simulink model "hethong_RR1"  (R2023a)
settings: Solver=FixedStepDiscrete  StartTime=0.0  StopTime=0  FixedStep=T_sample  RelTol=1e-3  EnableMultiTasking=on
values from neighbouring files (symbols this model uses):
  A = A_d    [GiaiBT_compactversion.m]    (also in KhoaModified_of_RLLQRroirac.m = [0        1.0047      0.0867      -0.0450; RLLQRroirac.m = [0        1.0047      0.0867      -0.0450; caithien_RLLQRroirac.m = [0        1.0047      0.0867      -0.0450)
  B = B_d    [GiaiBT_compactversion.m]    (also in KhoaModified_of_RLLQRroirac.m = [ 0.0450;    0.1038;    0.7378;    0.0007]; RLLQRroirac.m = [ 0.0450;    0.1038;    0.7378;    0.0007]; caithien_RLLQRroirac.m = [ 0.0450;    0.1038;    0.7378;    0.0007])
  D = D_d    [GiaiBT_compactversion.m]
  explore = rand    [GiaiBT_compactversion.m]    (also in KhoaModified_of_RLLQRroirac.m; RLLQRroirac.m; caithien_RLLQRroirac.m)
  K = H22\(H21')    [GiaiBT_compactversion.m]    (also in KhoaModified_of_RLLQRroirac.m = 1/(H22)*H21'; RLLQRroirac.m; caithien_RLLQRroirac.m = 1/(H22)*H21')
  x = [10;2.2]    [GiaiBT_compactversion.m]    (also in KhoaModified_of_RLLQRroirac.m = [0;0.1;0;0]; RLLQRroirac.m = [0;0.1;0;0]; caithien_RLLQRroirac.m = [0;0.1;0;0])
settings Model: Creator=Admin  LastModifiedBy=Admin
settings SolverCC: AlgebraicLoopSolver=TrustRegion
settings DataIOCC: LimitDataPoints=on  SaveFinalState=on  SaveFormat=Array  SignalLoggingSaveFormat=ModelDataLogs  ReturnWorkspaceOutputs=off
settings OptimizationCC: InitFltsAndDblsToZero=on  LifeSpan=inf
settings DebuggingCC: SaveWithParameterizedLinksMsg=none  UnderspecifiedInitializationDetection=Classic  MergeDetectMultiDrivingBlocksExec=none  SignalResolutionControl=TryResolveAllWithWarning  SolverPrmCheckMsg=warning  MultiTaskDSMMsg=warning  MultiTaskCondExecSysMsg=none  UnconnectedInputMsg=warning  UnconnectedOutputMsg=warning  UnconnectedLineMsg=warning  SFUnexpectedBacktrackingDiag=warning  SFNoUnconditionalDefaultTransitionDiag=warning  SFExecutionAtInitializationDiag=none  ArithmeticOperatorsInVariantConditions=warning
settings HardwareCC: ProdBitPerPointer=32  ProdBitPerSizeT=32  ProdBitPerPtrDiffT=32  ProdLargestAtomicFloat=None  ProdIntDivRoundTo=Undefined  ProdEndianess=Unspecified  ProdWordSize=32  ProdHWDeviceType=32-bit Generic
settings ModelReferenceCC: EnableRefExpFcnMdlSchedulingChecks=on  PropagateSignalLabelsOutOfModel=off
settings SFSimCC: CustomCodeUndefinedFunction=UseInterfaceOnly
settings CodeAppCC: StateflowObjectComments=on
settings GRTTargetCC: TargetFcnLib=ansi_tfl_tmw.mat  TargetLangStandard=C89/C90 (ANSI)  CombineOutputUpdateFcns=off  GRTInterface=on
settings ConfigComp: CovMetricSettings=dw  CovSaveCumulativeToWorkspaceVar=on  CovSaveSingleToWorkspaceVar=on

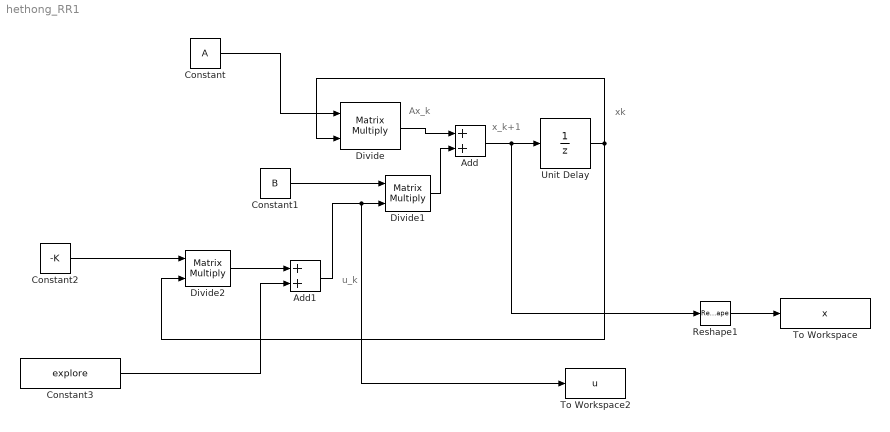
== system hethong_RR1 ==
  note: x_k+1
  note: u_k
  note: Ax_k
  note: xk
  Add : Sum
  Add1 : Sum
  Constant : Constant  Value=A  VectorParams1D=off
  Constant1 : Constant  Value=B  VectorParams1D=off
  Constant2 : Constant  Value=-K  VectorParams1D=off
  Constant3 : Constant  Value=explore  VectorParams1D=off
  Divide : Product  Inputs=**  Multiplication=Matrix(*)
  Divide1 : Product  Inputs=**  Multiplication=Matrix(*)
  Divide2 : Product  Inputs=**  Multiplication=Matrix(*)
  Reshape1 : Reshape  OutputDimensionality=Column vector (2-D)
  To Workspace : ToWorkspace  VariableName=x  SampleTime=-1
  To Workspace2 : ToWorkspace  VariableName=u  SampleTime=-1
      settings: MaxDataPoints=1
  Unit Delay : UnitDelay  InitialCondition=x  SampleTime=-1
  wires:
  Constant/1 -> Divide/1
  Constant1/1 -> Divide1/1
  Add/1 -> Reshape1/1, Unit Delay/1
  Unit Delay/1 -> Divide2/2, Divide/2
  Constant2/1 -> Divide2/1
  Divide/1 -> Add/1
  Divide1/1 -> Add/2
  Reshape1/1 -> To Workspace/1
  Divide2/1 -> Add1/1
  Add1/1 -> To Workspace2/1, Divide1/2
  Constant3/1 -> Add1/2
